simulink model "Frequency_Derivation"  (R2018a)
settings: Solver=VariableStepAuto  StartTime=0.0  StopTime=10.0  RelTol=1e-3
libraries: dspswit3 x1
settings Model: Creator=s249546  LastModifiedBy=s249546

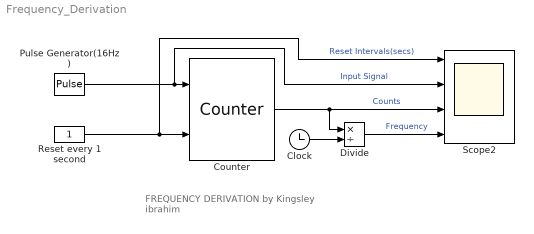
== system Frequency_Derivation ==
  note: FREQUENCY DERIVATION
      | by Kingsley ibrahim
  Clock : Clock
  Counter : dspswit3/Counter  Direction=Up  CountEvent=Rising edge  CounterSize=User defined  MaxCount=12000  InitialCount=0  Output=Count  HitValue=1  ResetInput=on  SamplesPerFrame=1  Ts=1  CntDtype=double  HitDtype=Logical
  Divide : Product  Inputs=*/
  Pulse Generator(16Hz) : DiscretePulseGenerator  PulseType=Time based  Period=1/16  PulseWidth=50
  Reset every 1 second : Constant
  Scope2 : Scope  NumInputPorts=4
  wires:
  Reset every 1 second/1 -> Scope2/1, Counter/2  "Reset Intervals(secs)"
  Clock/1 -> Divide/2
  Pulse Generator(16Hz)/1 -> Counter/1, Scope2/2  "Input Signal"
  Divide/1 -> Scope2/4  "Frequency"
  Counter/1 -> Scope2/3, Divide/1  "Counts"
